simulink model "differential_drive_kinematic"  (R2020b)
settings: Solver=ode1  StartTime=0.0  StopTime=inf  FixedStep=0.01  RelTol=1e-3
libraries: simulink x1
settings Model: Creator=ONLY-GOD  LastModifiedBy=ONLY-GOD

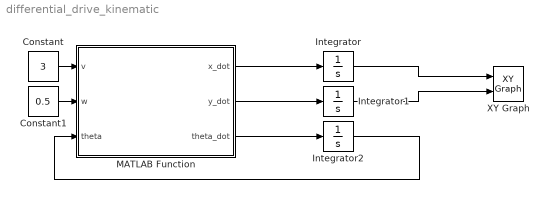
== system differential_drive_kinematic ==
  Constant : Constant  Value=3
  Constant1 : Constant  Value=0.5
  Integrator : Integrator
  Integrator1 : Integrator
  Integrator2 : Integrator
  MATLAB Function : MATLAB Function  TreatAsAtomicUnit=on
  XY Graph : simulink/Sinks/XY Graph  xmin=-5  xmax=5  ymin=-5  ymax=5  st=-1
  wires:
  Constant/1 -> MATLAB Function/1(v)
  Constant1/1 -> MATLAB Function/2(w)
  MATLAB Function/1(x_dot) -> Integrator/1
  MATLAB Function/2(y_dot) -> Integrator1/1
  MATLAB Function/3(theta_dot) -> Integrator2/1
  Integrator2/1 -> MATLAB Function/3(theta)
  Integrator/1 -> XY Graph/1
  Integrator1/1 -> XY Graph/2

== matlab function differential_drive_kinematic/MATLAB Function ==
  data: v input; x_dot output; w input; y_dot output; theta_dot output; theta input
function [x_dot,y_dot,theta_dot]= kinematic(v,w,theta)
x_dot = v*cos(theta);
y_dot = v*sin(theta);
theta_dot = w;
